simulink model "CodeGen_IP"  (R2021a)
settings: Solver=VariableStepAuto  StartTime=0.0  StopTime=10  RelTol=1e-3  EnableMultiTasking=on
undefined symbols (not defined in the file): A, AXI4, gray, N, Stream, video, xc7k325tffg900
libraries: hlsBasic x3, Sobeledge_lib x2, visionsinks x2, hlsUtilities x1, dspvision x1, vmcUtilities x1
settings Model: Creator=dvancamp  LastModifiedBy=robg
settings SolverCC: AlgebraicLoopSolver=TrustRegion
settings DataIOCC: LimitDataPoints=on  ReturnWorkspaceOutputs=off
settings OptimizationCC: LifeSpan=inf
settings DebuggingCC: InheritedTsInSrcMsg=none  AllowSymbolicDim=off  SFUnexpectedBacktrackingDiag=warning  SFNoUnconditionalDefaultTransitionDiag=warning  SFMachineParentedDataDiag=warning  ArithmeticOperatorsInVariantConditions=warning
settings ModelReferenceCC: PropagateSignalLabelsOutOfModel=off
settings SFSimCC: SimUseLocalCustomCode=off  CustomCodeUndefinedFunction=UseInterfaceOnly
settings RTWCC: RTWUseLocalCustomCode=off
settings CodeAppCC: StateflowObjectComments=on
settings GRTTargetCC: TargetLangStandard=C89/C90 (ANSI)
settings ConfigComp: CovMetricSettings=dw  CovSaveCumulativeToWorkspaceVar=on  CovSaveSingleToWorkspaceVar=on  CovExternalEMLEnable=off

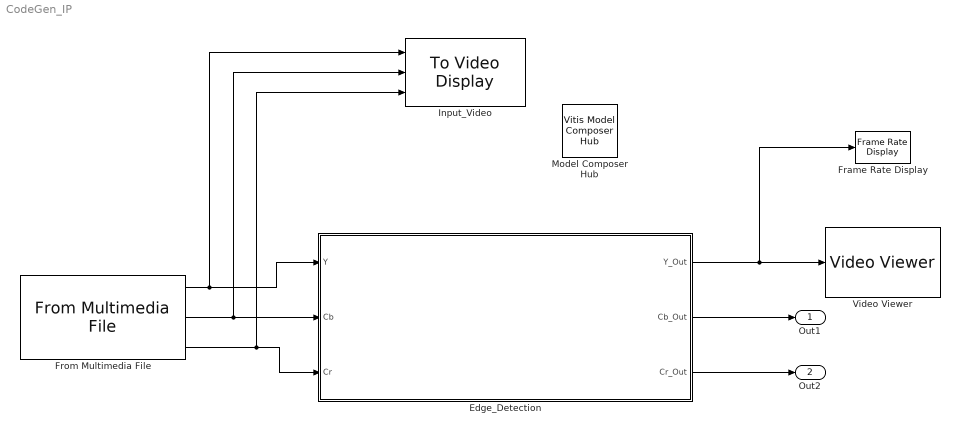
== system CodeGen_IP ==
  Edge_Detection : Subsystem
  Frame Rate Display : visionsinks/Frame Rate Display  UpdateRate=10
      settings: SourceProductBaseCode=VP
  From Multimedia File : dspvision/From Multimedia File  inputFilename=visiontraffic.avi  readRange=[1 Inf]  loop=on  numPlays=inf  outputStreams=Video only  videoDataType=uint8  audioDataType=int16  inheritSampleTime=off  userDefinedSampleTime=1/30  noAudioOutput=off  isIntensityVideo=off  fourcc=YCbCr 4:2:2  colorVideoFormat=Separate color signals  outputEOF=off  dataOrg=Column-major  audioFrameSize=1024  computeAudioFrameSize=off  outSamplingMode=Sample based
  Input_Video : visionsinks/To Video Display  windowSizeMode=Normal  openAtMdlStart=on  fullScreen=off  videoWindowX=150  videoWindowY=269  saveWindowSize=off  videoWindowWidth=581  videoWindowHeight=403  inputColorFormat=YCbCr 4:2:2  inputType=Obsolete  imagePorts=One multidimensional signal  OutputDevice=On-screen video monitor  dataOrg=Column-major  isWindowOpen=off
  Model Composer Hub : vmcUtilities/Vitis Model Composer Hub  Tag=genX  Description=Performs multiplication  CodeGeneration=off  SubsystemName=Edge_Detection  TargetDirectory=./codegen_IP  ExportType=IP Catalog  IpVendor=xilinx.com  IpLibrary=hls  IpName=Edge_Detection  IpVersion=1.0  IpHWLanguage=Verilog  AieCompilerOptions={}  CreateTestbench=off  TestbenchStackSize=10  RunAieSim=off  AieSimTimeout=50000  RunAieSimProfiling=off  LaunchVitisAnalyzer=off  PlotOutput=off  RunX86Sim=on  X86SimTimeout=10  GenHwImage=off  PlatformType=Not Specified  HwSystemType=Baremetal  HwValidationTarget=hw  ProjDevice=Kintex-7 KC705 Evaluation Platform (xc7k325tffg900-2)  ProjDevicePart=xc7k325tffg900-2  SamplePeriod=-1  ClockFrequency=200  DataPathParallelism=1  xilinxfamily=kintex7  part=xc7k325t  speed=-2  package=ffg900  directory=./netlist  testbench=off  incr_netlist=off  synthesis_tool=Vivado  clock_wrapper=Clock Enables  dbl_ovrd=According to Block Masks  dcm_input_clock_period=10  sysclk_period=10  simulink_period=1  eval_field=0  IPInfoJsonString="{\"HLSSubsystem\":{\"SubsystemName\":\"Edge_Detection\",\"IPName\":\"Edge_Detection\",\"IPLibrary\":\"hls\",\"IPVendor\":\"xilinx.com\",\"IPVersion\":\"1.0\"}}"
  Video Viewer : VideoViewer  colormapValue=gray(256)  FigPos=[755.4 765.2 589.6 316]
  Out1 : Outport
  Out2 : Outport  Port=2
  wires:
  From Multimedia File/1 -> Edge_Detection/1(Y), Input_Video/1
  Edge_Detection/1(Y_Out) -> Video Viewer/1, Frame Rate Display/1
  From Multimedia File/2 -> Input_Video/2, Edge_Detection/2(Cb)
  From Multimedia File/3 -> Input_Video/3, Edge_Detection/3(Cr)
  Edge_Detection/2(Cb_Out) -> Out1/1
  Edge_Detection/3(Cr_Out) -> Out2/1

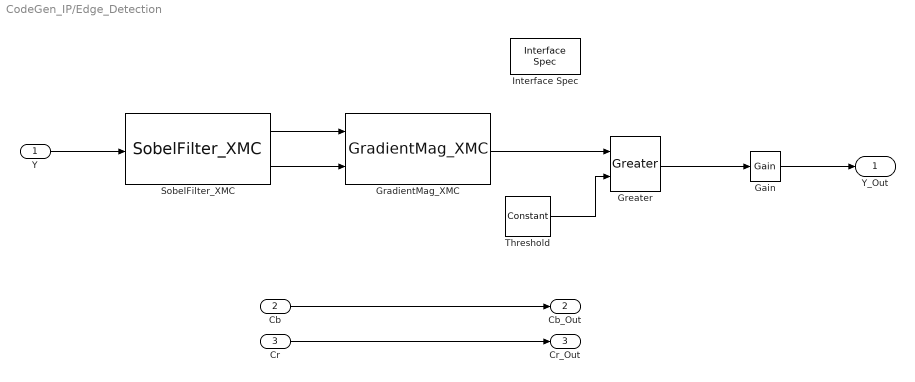
== system CodeGen_IP/Edge_Detection ==
  Y : Inport
  Cb : Inport  Port=2
  Cr : Inport  Port=3
  Gain : hlsBasic/Gain  Gain=255  OutDataType=uint8  TypeExp=''  Signedness=Signed  WordLength=16  FractionalLength=10  RoundingMode=Truncation to minus infinity  OverflowMode=Wrap around  OutputTypeAsInput=off
  GradientMag_XMC : Sobeledge_lib/GradientMag_XMC  LibraryFunction=GradientMag_XMC  IncludeFiles={'GradientMag_Wrap.h'}  SourceFiles={}  IncludeDirectories={'./include'}  TemplateParams={'int ROWS'; 'int COLS'; 'int NPC'}  FunctionParamTypes={xmcDataType('void'); xmcDataType('uint16_t'); xmcDataType('uint16_t'); xmcDataType('uint16_t'); xmcDataType('int')}  FunctionParamPassbys={0.000000000000000000e+00; 0.000000000000000000e+00; 0.000000000000000000e+00; 0.000000000000000000e+00; 0.000000000000000000e+00}  FunctionParamDimensions={'1'; '[ROWS][COLS]'; '[ROWS][COLS]'; '[ROWS][COLS]'; '1'}  FunctionParamNames={'return'; 'inX'; 'inY'; 'Out'; 'NPC'}  FunctionParamDir={0.000000000000000000e+00; 1.000000000000000000e+00; 1.000000000000000000e+00; 2.000000000000000000e+00; 3.000000000000000000e+00}  FunctionParamSupportsStreaming={true; true; true; true; true}  BufferDepth={'0'}  FunctionParamValues={'0'; '0'; '0'; '0'; '0'}  ThroughputFactors={''}  NPC=1
  Greater : hlsBasic/Greater  Description=Performs multiplication
  Interface Spec : hlsUtilities/Interface Spec  Return=AXI4-Lite Slave@@  InportInterfaces={'AXI4-Stream (video)@image_in@@YUV 4:2:2@Y', 'AXI4-Stream (video)@image_in@@YUV 4:2:2@U', 'AXI4-Stream (video)@image_in@@YUV 4:2:2@V'}  InportHandles={3.001464843750000000e+00, 4.001464843750000000e+00, 5.001464843750000000e+00}  InportNames={'Y', 'Cb', 'Cr'}  OutportInterfaces={'AXI4-Stream (video)@image_out@@YUV 4:2:2@Y', 'AXI4-Stream (video)@image_out@@YUV 4:2:2@U', 'AXI4-Stream (video)@image_out@@YUV 4:2:2@V'}  OutportHandles={1.200146484375000000e+01, 1.300146484375000000e+01, 1.400146484375000000e+01}  OutportNames={'Y_Out', 'Cb_Out', 'Cr_Out'}  Mode=AXI4-Lite Slave  InName1=Y  InMode1=AXI4-Stream (video)  InBundle1=image_in  InVFormat1=YUV 4:2:2  InVComponent1=Y  InName2=Cb  InMode2=AXI4-Stream (video)  InBundle2=image_in  InVFormat2=YUV 4:2:2  InVComponent2=U  InName3=Cr  InMode3=AXI4-Stream (video)  InBundle3=image_in  InVFormat3=YUV 4:2:2  InVComponent3=V  InMode4=Default  InVFormat4=N/A  InVComponent4=N/A  InMode5=Default  InVFormat5=N/A  InVComponent5=N/A  InMode6=Default  InVFormat6=N/A  InVComponent6=N/A  InMode7=Default  InVFormat7=N/A  InVComponent7=N/A  InMode8=Default  InVFormat8=N/A  InVComponent8=N/A  OutName1=Y_Out  OutMode1=AXI4-Stream (video)  OutBundle1=image_out  OutVFormat1=YUV 4:2:2  OutVComponent1=Y  OutName2=Cb_Out  OutMode2=AXI4-Stream (video)  OutBundle2=image_out  OutVFormat2=YUV 4:2:2  OutVComponent2=U  OutName3=Cr_Out  OutMode3=AXI4-Stream (video)  OutBundle3=image_out  OutVFormat3=YUV 4:2:2  OutVComponent3=V  OutMode4=Default  OutVFormat4=N/A  OutVComponent4=N/A  OutMode5=Default  OutVFormat5=N/A  OutVComponent5=N/A  OutMode6=Default  OutVFormat6=N/A  OutVComponent6=N/A  OutMode7=Default  OutVFormat7=N/A  OutVComponent7=N/A  OutMode8=Default  OutVFormat8=N/A  OutVComponent8=N/A
  SobelFilter_XMC : Sobeledge_lib/SobelFilter_XMC  LibraryFunction=SobelFilter_XMC  IncludeFiles={'sobelfilter_Wrap.h'}  SourceFiles={}  IncludeDirectories={'./include'}  TemplateParams={'int ROWS'; 'int COLS'; 'int NPC'}  FunctionParamTypes={xmcDataType('void'); xmcDataType('uint8_t'); xmcDataType('uint16_t'); xmcDataType('uint16_t'); xmcDataType('int')}  FunctionParamPassbys={0.000000000000000000e+00; 0.000000000000000000e+00; 0.000000000000000000e+00; 0.000000000000000000e+00; 0.000000000000000000e+00}  FunctionParamDimensions={'1'; '[ROWS][COLS]'; '[ROWS][COLS]'; '[ROWS][COLS]'; '1'}  FunctionParamNames={'return'; 'in'; 'outX'; 'outY'; 'NPC'}  FunctionParamDir={0.000000000000000000e+00; 1.000000000000000000e+00; 2.000000000000000000e+00; 2.000000000000000000e+00; 3.000000000000000000e+00}  FunctionParamSupportsStreaming={true; true; true; true; true}  BufferDepth={'0'}  FunctionParamValues={'0'; '0'; '0'; '0'; '0'}  ThroughputFactors={''}  NPC=1
  Threshold : hlsBasic/Constant  Description=Performs multiplication  Value=150  VectorParams1D=off  SampleTime=-1  OutDataType=int16  TypeExp=''  Signedness=Signed  WordLength=16  FractionalLength=0  RoundingMode=Truncation to minus infinity  OverflowMode=Wrap around
  Y_Out : Outport
  Cb_Out : Outport  Port=2
  Cr_Out : Outport  Port=3
  wires:
  Cb/1 -> Cb_Out/1
  Cr/1 -> Cr_Out/1
  Y/1 -> SobelFilter_XMC/1
  Threshold/1 -> Greater/2
  GradientMag_XMC/1 -> Greater/1
  SobelFilter_XMC/1 -> GradientMag_XMC/1
  SobelFilter_XMC/2 -> GradientMag_XMC/2
  Greater/1 -> Gain/1
  Gain/1 -> Y_Out/1
